simulink subsystem "spwm_switching"  (R2024a)
settings: Solver=VariableStepAuto  StartTime=0.0  StopTime=10.0  RelTol=1e-3
settings Model: Creator=javeed  LastModifiedBy=javeed

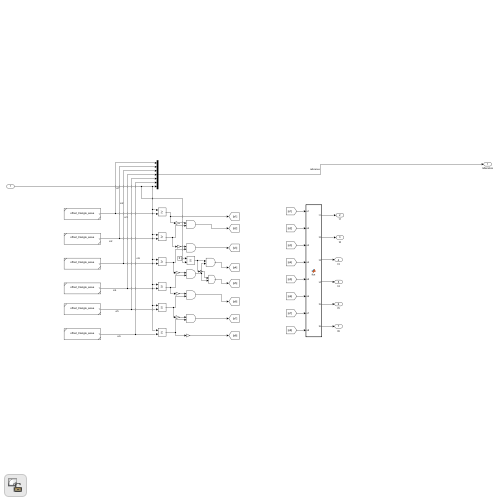
[thumbnail: Simulink's stored preview of the top-level diagram]
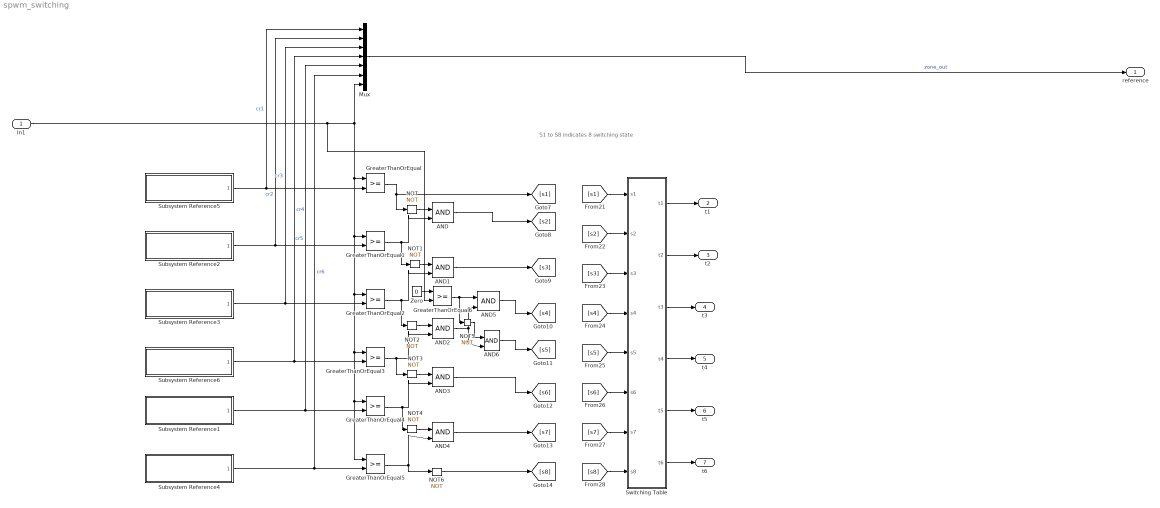
== system spwm_switching ==
  note: S1 to S8 indicates 8 switching state
  In1 : Inport
  AND{,1..6} (7 alike) : Logic  IconShape=distinctive  AllPortsSameDT=off  OutDataTypeStr=boolean
  GreaterThanOrEqual{,1..4,6} (6 alike) : RelationalOperator  OutDataTypeStr=boolean  RndMeth=Simplest  InputSameDT=off
  GreaterThanOrEqual5 : RelationalOperator  OutDataTypeStr=fixdt(0,1,0)  RndMeth=Simplest  InputSameDT=off
  Mux : Mux  Inputs=7
  NOT{,1..6} (7 alike) : Logic  Operator=NOT  IconShape=distinctive  AllPortsSameDT=off  OutDataTypeStr=boolean
  Subsystem Reference1 : Subsystem  ReferencedSubsystem=offset_triangle_wave  offset=-3/6  gain=1/6  freq=switching_freq
  Subsystem Reference2 : Subsystem  ReferencedSubsystem=offset_triangle_wave  offset=3/6  gain=1/6  freq=switching_freq
  Subsystem Reference3 : Subsystem  ReferencedSubsystem=offset_triangle_wave  offset=1/6  gain=1/6  freq=switching_freq
  Subsystem Reference4 : Subsystem  ReferencedSubsystem=offset_triangle_wave  offset=-5/6  gain=1/6  freq=switching_freq
  Subsystem Reference5 : Subsystem  ReferencedSubsystem=offset_triangle_wave  offset=5/6  gain=1/6  freq=switching_freq
  Subsystem Reference6 : Subsystem  ReferencedSubsystem=offset_triangle_wave  offset=-1/6  gain=1/6  freq=switching_freq
  Switching Table : MATLAB Function  Description=|  TreatAsAtomicUnit=on
      | This block act as an encoder for switching state. It will give corresponding switching Signal for the switches(T1 - T6) for States S1 to S8.
      | Chat gpt this coe for understanding
  Zero : Constant  Value=0  OutDataTypeStr=Inherit: Inherit via back propagation
  reference : Outport
  t1 : Outport  Port=2
  t2 : Outport  Port=3
  t3 : Outport  Port=4
  t4 : Outport  Port=5
  t5 : Outport  Port=6
  t6 : Outport  Port=7
  wires:
  Zero/1 -> GreaterThanOrEqual6/1
  Subsystem Reference5/1 -> GreaterThanOrEqual/2, Mux/1  "cr1"
  NOT5/1 -> AND6/1
  GreaterThanOrEqual6/1 -> NOT5/1, AND5/1
  Subsystem Reference2/1 -> Mux/2, GreaterThanOrEqual1/2  "cr2"
  GreaterThanOrEqual3/1 -> NOT3/1, AND2/2
  [s6] -> Switching Table/6(s6)
  Subsystem Reference4/1 -> Mux/6, GreaterThanOrEqual5/2  "cr6"
  NOT2/1 -> AND2/1
  In1/1 -> Mux/7, GreaterThanOrEqual/1, GreaterThanOrEqual1/1, GreaterThanOrEqual2/1, GreaterThanOrEqual3/1, GreaterThanOrEqual4/1, GreaterThanOrEqual5/1, GreaterThanOrEqual6/2
  GreaterThanOrEqual2/1 -> AND1/2, NOT2/1
  GreaterThanOrEqual1/1 -> AND/2, NOT1/1
  AND6/1 -> [s5]
  GreaterThanOrEqual4/1 -> AND3/2, NOT4/1
  [s2] -> Switching Table/2(s2)
  AND5/1 -> [s4]
  NOT4/1 -> AND4/1
  GreaterThanOrEqual5/1 -> AND4/2, NOT6/1
  AND1/1 -> [s3]
  GreaterThanOrEqual/1 -> [s1], NOT/1
  AND3/1 -> [s6]
  [s3] -> Switching Table/3(s3)
  NOT3/1 -> AND3/1
  AND4/1 -> [s7]
  NOT6/1 -> [s8]
  AND2/1 -> AND6/2, AND5/2
  Subsystem Reference3/1 -> Mux/3, GreaterThanOrEqual2/2  "cr3"
  Subsystem Reference6/1 -> Mux/4, GreaterThanOrEqual3/2  "cr4"
  NOT1/1 -> AND1/1
  Subsystem Reference1/1 -> Mux/5, GreaterThanOrEqual4/2  "cr5"
  [s7] -> Switching Table/7(s7)
  [s8] -> Switching Table/8(s8)
  AND/1 -> [s2]
  Switching Table/5(t5) -> t5/1
  [s5] -> Switching Table/5(s5)
  Switching Table/3(t3) -> t3/1
  [s4] -> Switching Table/4(s4)
  NOT/1 -> AND/1
  [s1] -> Switching Table/1(s1)
  Mux/1 -> reference/1  "zone_out"
  Switching Table/4(t4) -> t4/1
  Switching Table/1(t1) -> t1/1
  Switching Table/2(t2) -> t2/1
  Switching Table/6(t6) -> t6/1

== matlab function spwm_switching/Switching Table ==
  data: s1 input; t1 output; s2 input; s3 input; s4 input; s5 input; s6 input; s7 input; s8 input; t2 output; t3 output; t4 output; t5 output; t6 output
function [t1,t2,t3,t4,t5,t6] = fcn(s1,s2,s3,s4,s5,s6,s7,s8)
    % Define the state matrix from the inputs
    state_mat = [s1,s2,s3,s4,s5,s6,s7,s8];
    
    % Define the switching table
    switching_table = [
        1 0 1 0 1 0;
        1 0 0 0 1 1;
        0 0 1 1 1 0;
        0 0 0 1 1 1;
        1 1 1 0 0 0;
        1 1 0 0 0 1;
        0 1 1 1 0 0;
        0 1 0 1 0 1;
    ];
    switching_table = logical(switching_table);
    % Define a mapping from state_mat to row indices in the switching table
    state_map = [
        [1 0 0 0 0 0 0 0]; % state 1
        [0 1 0 0 0 0 0 0]; % state 2
        [0 0 1 0 0 0 0 0]; % state 3
        [0 0 0 1 0 0 0 0]; % state 4
        [0 0 0 0 1 0 0 0]; % state 5
        [0 0 0 0 0 1 0 0]; % state 6
        [0 0 0 0 0 0 1 0]; % state 7
        [0 0 0 0 0 0 0 1]; % state 8
    ];
    
    % Initialize output variables
    t1 = false;
    t2 = false;
    t3 = false;
    t4 = false;
    t5 = false;
    t6 = false;
    
    % Loop through the state_map to find the correct state index
    for i = 1:size(state_map, 1)
        if isequal(state_mat, state_map(i,:))
            % Get the row from the switching_table based on the state index
            row = switching_table(i, :);
            % Assign the values to the output variables
            [t1, t2, t3, t4, t5, t6] = deal(row(1), row(2), row(3), row(4), row(5), row(6));
            return;
        end
    end
end
